simulink model "our_linear_mpc"  (R2024b)
settings: Solver=ode4  StartTime=0.0  StopTime=10  FixedStep=0.02  RelTol=1e-3
settings Model: Creator=Manuela  LastModifiedBy=kaiqu

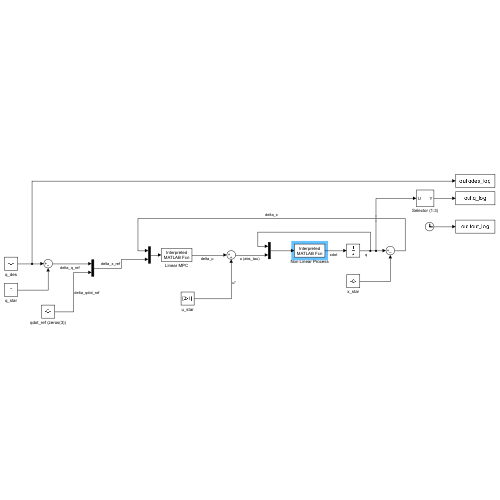
[thumbnail: Simulink's stored preview of the top-level diagram]
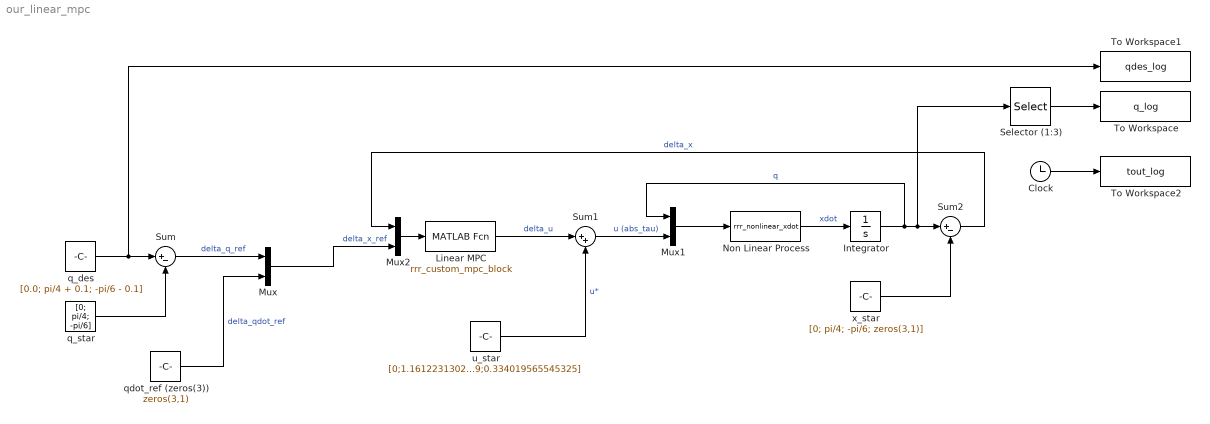
== system our_linear_mpc ==
  Clock : Clock
  Integrator : Integrator  InitialCondition=[0; pi/4; -pi/6; zeros(3,1)]
  Linear MPC : MATLABFcn  MATLABFcn=rrr_custom_mpc_block
  Mux : Mux  Inputs=2
  Mux1 : Mux  Inputs=2
  Mux2 : Mux  Inputs=2
  Non Linear Process : MATLABFcn  MATLABFcn=rrr_nonlinear_xdot  OutputDimensions=6
  Selector (1:3) : Selector  InputPortWidth=6  IndexOptions=Index vector (dialog)  Indices=[1 2 3]  OutputSizes=1
  Sum : Sum  Inputs=|+-
  Sum1 : Sum  Inputs=|++
  Sum2 : Sum  Inputs=|+-
  To Workspace : ToWorkspace  VariableName=q_log  SampleTime=-1
  To Workspace1 : ToWorkspace  VariableName=qdes_log  SampleTime=0.02
  To Workspace2 : ToWorkspace  VariableName=tout_log  SampleTime=-1
  q_des : Constant  Tag=q_des  Description=q_des  Value=[0.0; pi/4 + 0.1; -pi/6 - 0.1]  SampleTime=0.02
  q_star : Constant  Value=[0; pi/4; -pi/6]
  qdot_ref (zeros(3)) : Constant  Value=zeros(3,1)
  u_star : Constant  Value=[0;1.161223130215549;0.334019565545325]
  x_star : Constant  Value=[0; pi/4; -pi/6; zeros(3,1)]
  wires:
  q_des/1 -> To Workspace1/1, Sum/1
  q_star/1 -> Sum/2
  Sum/1 -> Mux/1  "delta_q_ref"
  qdot_ref (zeros(3))/1 -> Mux/2  "delta_qdot_ref"
  Mux/1 -> Mux2/2  "delta_x_ref"
  Linear MPC/1 -> Sum1/1  "delta_u"
  u_star/1 -> Sum1/2  "u*"
  Non Linear Process/1 -> Integrator/1  "xdot"
  x_star/1 -> Sum2/2
  Integrator/1 -> Selector (1:3)/1, Sum2/1, Mux1/1  "q"
  Sum1/1 -> Mux1/2  "u (abs_tau)"
  Mux1/1 -> Non Linear Process/1
  Sum2/1 -> Mux2/1  "delta_x"
  Selector (1:3)/1 -> To Workspace/1
  Clock/1 -> To Workspace2/1
  Mux2/1 -> Linear MPC/1
